simulink model "s_tanks_1_id"  (R2021a)
settings: Solver=ode4  StartTime=0.0  StopTime=6000  FixedStep=0.002  RelTol=1e-3  EnableMultiTasking=on
undefined symbols (not defined in the file or in its folder): Ao1, At1, g, Kp, VMAX_AMP
libraries: slident x1
settings Model: ExtModeTrigDuration=30000  Creator=MLevis  LastModifiedBy=tronc
settings SolverCC: AlgebraicLoopSolver=TrustRegion  PositivePriorityOrder=on
settings DataIOCC: LimitDataPoints=on  SaveFormat=Array  SignalLoggingSaveFormat=ModelDataLogs  ReturnWorkspaceOutputs=off
settings OptimizationCC: ExpressionDepthLimit=2147483647  InitFltsAndDblsToZero=on  LifeSpan=inf
settings DebuggingCC: SaveWithParameterizedLinksMsg=none  UnderspecifiedInitializationDetection=Classic  MergeDetectMultiDrivingBlocksExec=none  SolverPrmCheckMsg=warning  FcnCallInpInsideContextMsg=warning  StateNameClashWarn=warning  SFUnexpectedBacktrackingDiag=warning  SFNoUnconditionalDefaultTransitionDiag=warning  SFExecutionAtInitializationDiag=none  SFMachineParentedDataDiag=warning  ArithmeticOperatorsInVariantConditions=warning
settings HardwareCC: ProdBitPerPointer=32  ProdBitPerSizeT=32  ProdBitPerPtrDiffT=32  ProdLargestAtomicFloat=None  ProdIntDivRoundTo=Undefined  ProdEndianess=Unspecified  ProdWordSize=32  ProdHWDeviceType=32-bit Generic
settings ModelReferenceCC: PropagateSignalLabelsOutOfModel=off
settings RTWCC: Description=QuaRC Win32 Target  SystemTargetFile=quarc_windows.tlc  TemplateMakefile=quarc_default_tmf
settings CodeAppCC: StateflowObjectComments=on
settings STFCustomTargetCC: TargetFcnLib=ansi_tfl_tmw.mat  TargetPreCompLibLocation=C:\DOCUME~1\ALLUSE~1\APPLIC~1\QUARC\lib\2007b\windows\release  CPPClassGenCompliant=on  UseToolchainInfoCompliant=off  SystemTargetFile=quarc_windows.tlc
settings GRTTargetCC: TargetFcnLib=ansi_tfl_tmw.mat  TargetPreCompLibLocation=C:\DOCUME~1\ALLUSE~1\APPLIC~1\QUARC\lib\2007b\windows\release  TargetLangStandard=C89/C90 (ANSI)  ParMdlRefBuildCompliant=off  CompOptLevelCompliant=off  ConcurrentExecutionCompliant=off  CombineOutputUpdateFcns=off  MatFileLogging=off  GRTInterface=on  UseToolchainInfoCompliant=off  ExtMode=on  ExtModeMexFile=quarc_comm
settings ConfigComp: CovMetricSettings=dw  CovSaveCumulativeToWorkspaceVar=on  CovSaveSingleToWorkspaceVar=on

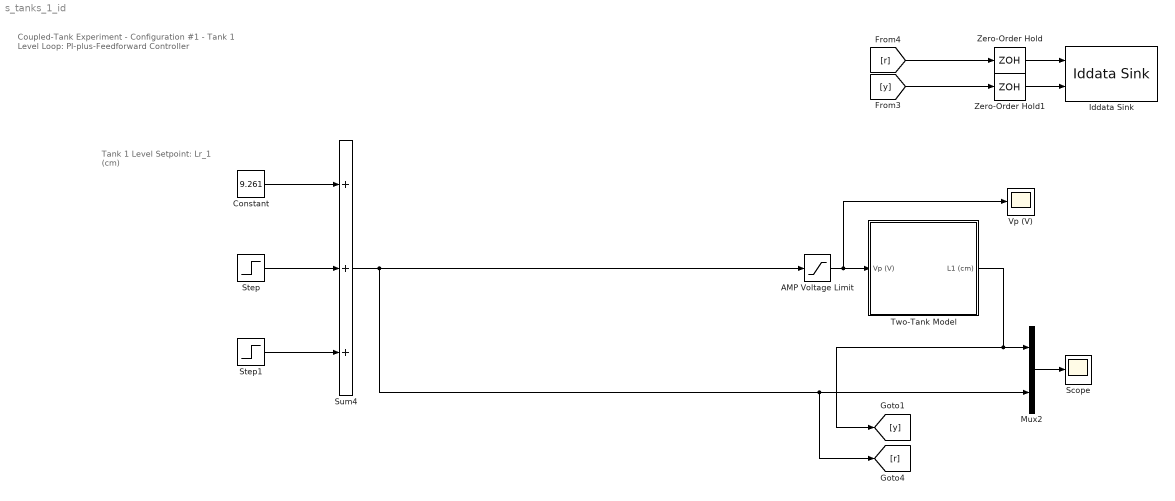
== system s_tanks_1_id ==
  note: Coupled-Tank Experiment
      | - Configuration #1 -
      | Tank 1 Level Loop:
      | PI-plus-Feedforward Controller
  note: Tank 1 Level Setpoint:
      | Lr_1 (cm)
  AMP Voltage Limit : Saturate  UpperLimit=VMAX_AMP  LowerLimit=0
  Constant : Constant  Value=9.261
  Iddata Sink : slident/Iddata Sink  datasetname=data_1  Ts=0.1  isu=on  isy=on
      settings: SourceProductBaseCode=ID
  Mux2 : Mux  Inputs=2
  Scope : Scope
  Step : Step  Time=2000  After=0.302  SampleTime=0
  Step1 : Step  Time=4000  After=-0.615  SampleTime=0
  Sum4 : Sum  Inputs=+++  InputSameDT=on  SaturateOnIntegerOverflow=on  OutDataTypeStr=Inherit: Same as first input
  Two-Tank Model : Subsystem
  "Vp (V) " : Scope
  Zero-Order Hold : ZeroOrderHold  SampleTime=0.1
  Zero-Order Hold1 : ZeroOrderHold  SampleTime=0.1
  wires:
  Mux2/1 -> Scope/1
  AMP Voltage Limit/1 -> Two-Tank Model/1(Vp (V)), "Vp (V) "/1
  Sum4/1 -> AMP Voltage Limit/1, [r], Mux2/2
  Two-Tank Model/1(L1 (cm)) -> [y], Mux2/1
  Constant/1 -> Sum4/1
  Zero-Order Hold1/1 -> Iddata Sink/2
  [r] -> Zero-Order Hold/1
  Zero-Order Hold/1 -> Iddata Sink/1
  [y] -> Zero-Order Hold1/1
  Step1/1 -> Sum4/3
  Step/1 -> Sum4/2

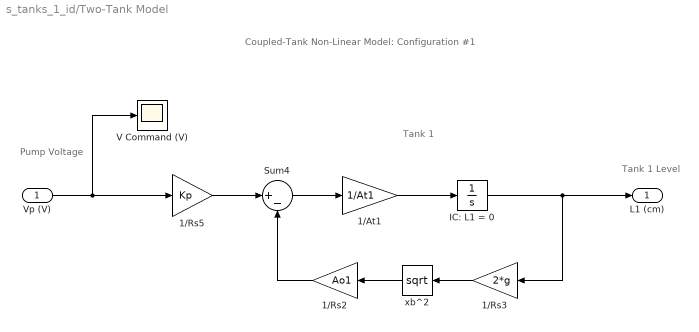
== system s_tanks_1_id/Two-Tank Model ==
  note: Coupled-Tank Non-Linear Model:
      | Configuration #1
  note: Tank 1
  note: Tank 1 Level
  note: Pump
      | Voltage
  Vp (V) : Inport
  1/At1 : Gain  Gain=1/At1  SaturateOnIntegerOverflow=on  OutDataTypeStr=Inherit: Same as input  ParamDataTypeStr=Inherit: Same as input
  1/Rs2 : Gain  Gain=Ao1  SaturateOnIntegerOverflow=on  OutDataTypeStr=Inherit: Same as input  ParamDataTypeStr=Inherit: Same as input
  1/Rs3 : Gain  Gain=2*g  SaturateOnIntegerOverflow=on  OutDataTypeStr=Inherit: Same as input  ParamDataTypeStr=Inherit: Same as input
  1/Rs5 : Gain  Gain=Kp  SaturateOnIntegerOverflow=on  OutDataTypeStr=Inherit: Same as input  ParamDataTypeStr=Inherit: Same as input
  IC: L1 = 0 : Integrator
  Sum4 : Sum  Inputs=|+-  InputSameDT=on  SaturateOnIntegerOverflow=on  OutDataTypeStr=Inherit: Same as first input
  V Command (V) : Scope
  xb^2 : Math  Operator=sqrt  SignedPower=on  SaturateOnIntegerOverflow=on
  L1 (cm) : Outport  InitialOutput=0
  wires:
  Vp (V)/1 -> V Command (V)/1, 1/Rs5/1
  1/Rs5/1 -> Sum4/1
  Sum4/1 -> 1/At1/1
  1/At1/1 -> IC: L1 = 0/1
  IC: L1 = 0/1 -> 1/Rs3/1, L1 (cm)/1
  1/Rs2/1 -> Sum4/2
  xb^2/1 -> 1/Rs2/1
  1/Rs3/1 -> xb^2/1
